simulink model "PCtest_pLBase"  (R2021b)
settings: Solver=FixedStepAuto  StartTime=0.0  StopTime=600  FixedStep=0.005  RelTol=1e-3
libraries: PuppyLibrary x2
settings Model: Creator=kboxi  LastModifiedBy=kboxi

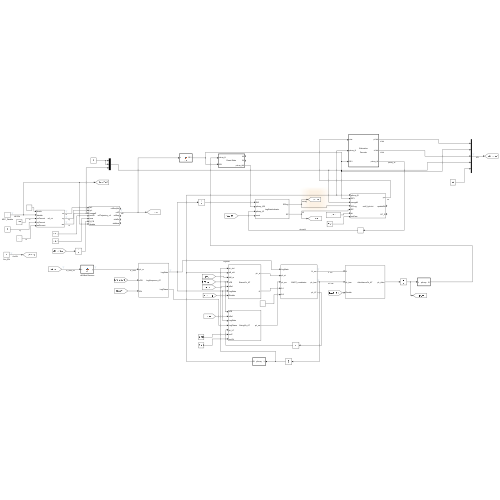
[thumbnail: Simulink's stored preview of the top-level diagram]
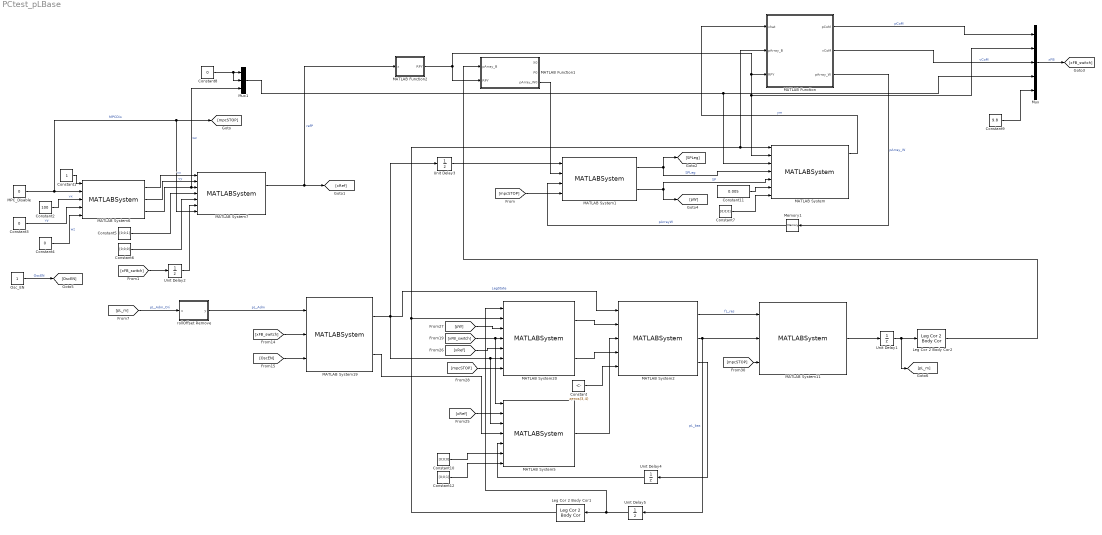
== system PCtest_pLBase ==
  Constant : Constant  Value=zeros(3,4)
  Constant1 : Constant
  Constant10 : Constant  Value=[0;0;0]
  Constant11 : Constant  Value=0.005
  Constant12 : Constant  Value=[0;0;1]
  Constant2 : Constant  Value=100
  Constant3 : Constant  Value=0
  Constant4 : Constant  Value=0
  Constant5 : Constant  Value=[0;0;1]
  Constant6 : Constant  Value=[0;0;0]
  Constant7 : Constant  Value=[0;0;0]
  Constant8 : Constant  Value=0
  Constant9 : Constant  Value=9.8
  Leg Cor 2 Body Cor1 : PuppyLibrary/Leg Cor 2 Body Cor  SystemSampleTime=-1  VariantActivationTime=update diagram  Latency=0  AutoFrameSizeCalculation=off
  Leg Cor 2 Body Cor2 : PuppyLibrary/Leg Cor 2 Body Cor  SystemSampleTime=-1  VariantActivationTime=update diagram  Latency=0  AutoFrameSizeCalculation=off
  MATLAB Function : MATLAB Function  TreatAsAtomicUnit=on
  MATLAB Function1 : MATLAB Function  TreatAsAtomicUnit=on
  MATLAB Function2 : MATLAB Function  TreatAsAtomicUnit=on
  MATLAB System : MATLABSystem  System=estX_byJoint  SimulateUsing=Code generation
      mask Type: estX_byJoint
      mask Display:
      | disp('estX_byJoint');
      | port_label('input',1,'pArray_B');
      | port_label('input',2,'RPY');
      | port_label('input',3,'omegaB');
      | port_label('input',4,'SPLeg');
      | port_label('input',5,'SP');
      | port_label('input',6,'dt');
      | port_label('input',7,'surPara');
      | port_label('output',1,'ym');
      | port_label('output',2,'updateEN');
      | port_label('output',3,'KF_R');
  MATLAB System1 : MATLABSystem  System=LegStateIndicator  SimulateUsing=Code generation
      mask Type: LegStateIndicator
      mask Display:
      | disp('LegStateIndicator');
      | port_label('input',1,'SW');
      | port_label('input',2,'pArray_W0');
      | port_label('input',3,'pArray_W');
      | port_label('input',4,'reset');
      | port_label('output',1,'SPLeg');
      | port_label('output',2,'SP');
  MATLAB System11 : MATLABSystem  System=AdmittanceCtr_AT  lateral_width=0.097  sagetial_width=0.2108  roll_Off=0.037  hIni=0.19  m=3  ks1=21  ks2=21  ks3=21  bs1=0  bs2=0  bs3=0  dt=0.005  SimulateUsing=Interpreted execution
      mask Type: AdmittanceCtr_AT
      mask Display:
      | disp('AdmittanceCtr_AT');
      | port_label('input',1,'fL');
      | port_label('input',2,'pL_bas');
      | port_label('input',3,'Disable');
      | port_label('output',1,'pL_Adm');
  MATLAB System19 : MATLABSystem  System=LegSequence_AT  tSW=0.3  SampleTime=0.005  OffsetTime=0  TickTime=0  startPhase=0  SimulateUsing=Interpreted execution
      mask Type: LegSequence_AT
      mask Display:
      | disp('LegSequence_AT');
      | port_label('input',1,'pL_m');
      | port_label('input',2,'xFB');
      | port_label('input',3,'EN');
      | port_label('output',1,'LegState');
      | port_label('output',2,'LegPhase');
  MATLAB System2 : MATLABSystem  System=SWST_combinator  SimulateUsing=Code generation
      mask Type: SWST_combinator
      mask Display:
      | disp('SWST_combinator');
      | port_label('input',1,'LegState');
      | port_label('input',2,'pL_st');
      | port_label('input',3,'pL_sw');
      | port_label('input',4,'fL1');
      | port_label('input',5,'fL2');
      | port_label('output',1,'fL_res');
      | port_label('output',2,'pL_bas');
      | port_label('output',3,'pL_LF');
  MATLAB System20 : MATLABSystem  System=StanceCtr_AT  tSW=0.3  tSample=0.005  r0=0.19  lateral_width=0.097  sagetial_width=0.2108  roll_Off=0.037  kp=zeros( 1, 6 )  kd=zeros( 1, 6 )  ki=zeros( 1, 6 )  SimulateUsing=Code generation
      mask Type: StanceCtr_AT
      mask Display:
      | disp('StanceCtr_AT');
      | port_label('input',1,'pL_old');
      | port_label('input',2,'pB_old');
      | port_label('input',3,'pW_m');
      | port_label('input',4,'xFB');
      | port_label('input',5,'xRef');
      | port_label('input',6,'LegState');
      | port_label('input',7,'Disable');
      | port_label('output',1,'pL_st');
      | port_label('output',2,'fL');
  MATLAB System5 : MATLABSystem  System=SwingCtr_AT  tSW=0.3  tSample=0.005  r0=[0;0;0.19]  StepH=0.05  lateral_width=0.097  sagetial_width=0.2108  roll_Off=0.037  kx_cv=0  kx_dv=0  ky_cv=0  ky_dv=0  k_wz=0.8  SimulateUsing=Code generation
      mask Type: SwingCtr_AT
      mask Display:
      | disp('SwingCtr_AT');
      | port_label('input',1,'xFB');
      | port_label('input',2,'xRef');
      | port_label('input',3,'LegState');
      | port_label('input',4,'LegPhase');
      | port_label('input',5,'pL_LF');
      | port_label('input',6,'surP');
      | port_label('input',7,'surVN');
      | port_label('output',1,'pL_sw');
  MATLAB System6 : MATLABSystem  System=ref_ctr  vxMax=0.3  vyMax=0.2  wzMax=0.8  SimulateUsing=Code generation
      mask Type: ref_ctr
      mask Display:
      | disp('ref_ctr');
      | port_label('input',1,'timeIn');
      | port_label('input',2,'disable');
      | port_label('input',3,'vxPercent');
      | port_label('input',4,'vyPercent');
      | port_label('input',5,'wzPercent');
      | port_label('output',1,'vx');
      | port_label('output',2,'vy');
      | port_label('output',3,'wz');
  MATLAB System7 : MATLABSystem  System=refTrajectory_v4  r0=[ 0; 0; 0.19 ]  theta0=[ 0; 0; 0 ]  dr0=[ 0; 0; 0 ]  omega0=[ 0; 0; 0 ]  desHeight=0.19  sitaErr_K=[0;0;0]  dt=0.005  numP=6  SimulateUsing=Code generation
      mask Type: refTrajectory_v4
      mask Display:
      | disp('refTrajectory_v4');
      | port_label('input',1,'vxL');
      | port_label('input',2,'vyL');
      | port_label('input',3,'omegaZ');
      | port_label('input',4,'surVN');
      | port_label('input',5,'sura');
      | port_label('input',6,'X_FB');
      | port_label('input',7,'disable');
      | port_label('output',1,'refSeqOut');
      | port_label('output',2,'refP');
      | port_label('output',3,'refSeq');
      | port_label('output',4,'sitaErr');
      | port_label('output',5,'sitaNow');
  MPC_Disable : Constant  Value=0
  Memory1 : Memory  InitialCondition=zeros(12,1)  InheritSampleTime=on
  Mux : Mux  Inputs=5
  Mux1 : Mux  Inputs=3
  Osc_EN : Constant
  Unit Delay1 : UnitDelay  InitialCondition=[0;0;-0.19;0;0;-0.19;0;0;-0.19;0;0;-0.19]*1000  SampleTime=-1  HasFrameUpgradeWarning=on
  Unit Delay2 : UnitDelay  InitialCondition=[0;0;0.19;zeros(9,1);9.8]  SampleTime=-1  HasFrameUpgradeWarning=on
  Unit Delay3 : UnitDelay  InitialCondition=[1;1;1;1]  SampleTime=-1  HasFrameUpgradeWarning=on
  Unit Delay4 : UnitDelay  InitialCondition=[0;0;-0.19;0;0;-0.19;0;0;-0.19;0;0;-0.19]  SampleTime=-1  HasFrameUpgradeWarning=on
  Unit Delay5 : UnitDelay  InitialCondition=[0;0;-0.19;0;0;-0.19;0;0;-0.19;0;0;-0.19]  SampleTime=-1  HasFrameUpgradeWarning=on
  rollOffset Remove : MATLAB Function  TreatAsAtomicUnit=on
  wires:
  [mpcSTOP] -> MATLAB System11/3
  MATLAB System2/1 -> MATLAB System11/1  "fL_res"
  Leg Cor 2 Body Cor1/1 -> MATLAB System20/2, MATLAB Function/2(pArray_B), MATLAB System/1
  Constant/1 -> MATLAB System2/5
  [xFB_switch] -> MATLAB System20/4, MATLAB System5/1
  MATLAB System2/2 -> MATLAB System11/2, Unit Delay5/1  "pL_bas"
  [xRef] -> MATLAB System5/2
  Unit Delay4/1 -> MATLAB System5/5
  MATLAB System2/3 -> Unit Delay4/1
  [OscEN] -> MATLAB System19/3
  MATLAB System20/2 -> MATLAB System2/4
  MATLAB System19/2 -> MATLAB System5/4
  [pW] -> MATLAB System20/3
  Unit Delay5/1 -> MATLAB System20/1, Leg Cor 2 Body Cor1/1
  MATLAB System20/1 -> MATLAB System2/2
  [mpcSTOP] -> MATLAB System20/7
  [xRef] -> MATLAB System20/5
  MATLAB System5/1 -> MATLAB System2/3
  MATLAB System19/1 -> MATLAB System2/1, Unit Delay3/1, MATLAB System20/6, MATLAB System5/3  "LegState"
  MPC_Disable/1 -> [mpcSTOP], MATLAB System7/7, MATLAB System6/2  "MPCDis"
  Constant1/1 -> MATLAB System6/1
  Constant2/1 -> MATLAB System6/3  "vx"
  Constant3/1 -> MATLAB System6/4  "vy"
  Constant4/1 -> MATLAB System6/5  "wz"
  MATLAB System6/1 -> MATLAB System7/1  "vx"
  MATLAB System6/2 -> MATLAB System7/2  "vy"
  MATLAB System6/3 -> Mux1/3, MATLAB System7/3  "wz"
  Constant5/1 -> MATLAB System7/4
  Constant6/1 -> MATLAB System7/5
  Memory1/1 -> MATLAB System1/3  "pArrayW"
  MATLAB Function/3(pArray_W) -> Memory1/1  "pArray_W"
  Constant11/1 -> MATLAB System/6
  MATLAB System1/1 -> [SPLeg], MATLAB System/4  "SPLeg"
  MATLAB System1/2 -> MATLAB System/5, [pW]  "SP"
  [mpcSTOP] -> MATLAB System1/4
  MATLAB System/1 -> MATLAB Function/1(xhat)  "ym"
  MATLAB Function1/3(pArray_W0) -> MATLAB System1/2
  MATLAB System7/2 -> [xRef], MATLAB Function2/1(x)  "refP"
  MATLAB Function2/1(RPY) -> MATLAB Function1/2(RPY), Mux/2, MATLAB System/2, MATLAB Function/3(RPY)
  Constant7/1 -> MATLAB System/7
  MATLAB Function/1(pCoM) -> Mux/1  "pCoM"
  MATLAB Function/2(vCoM) -> Mux/3  "vCoM"
  Constant8/1 -> Mux1/2, Mux1/1
  Mux1/1 -> MATLAB System/3, Mux/4
  Mux/1 -> [xFB_switch]  "xFB"
  Osc_EN/1 -> [OscEN]  "OscEN"
  Unit Delay1/1 -> [pL_m], Leg Cor 2 Body Cor2/1
  MATLAB System11/1 -> Unit Delay1/1
  Leg Cor 2 Body Cor2/1 -> MATLAB Function1/1(pArray_B)
  [xFB_switch] -> Unit Delay2/1
  Unit Delay2/1 -> MATLAB System7/6
  Constant9/1 -> Mux/5
  Constant10/1 -> MATLAB System5/6
  Constant12/1 -> MATLAB System5/7
  [xFB_switch] -> MATLAB System19/2
  Unit Delay3/1 -> MATLAB System1/1
  [pL_m] -> rollOffset Remove/1(u)  "pL_Adm_Ori"
  rollOffset Remove/1(y) -> MATLAB System19/1  "pL_Adm"

== matlab function PCtest_pLBase/rollOffset Remove ==
  data: u input; y output size=[12,1]
function y = fcn(u)
roll_Off=0.037;
tmp = reshape(u,3,4)-[0,0,0,0;
                    roll_Off,-roll_Off,roll_Off,-roll_Off;
                    0,0,0,0]*1000;
y=reshape(tmp,12,1)/1000;

== matlab function PCtest_pLBase/MATLAB Function2 ==
  data: x input; RPY output size=[3,1]
function RPY = fcn(x)
RPY=x(4:6);

== matlab function PCtest_pLBase/MATLAB Function ==
  data: xhat input; pCoM output size=[3,1]; vCoM output size=[3,1]; pArray_B input; RPY input; pArray_W output size=[12,1]
function [pCoM,vCoM,pArray_W] = fcn(xhat,pArray_B,RPY)
% pB the CoM position in the world coordinate
% vB the CoM velocity
% Wpi the foot-end position in the world coordinate
pCoM=[xhat(1);xhat(2);xhat(3)];
vCoM=[xhat(4);xhat(5);xhat(6)];
Rz=[cos(RPY(3)),-sin(RPY(3)),0;
    sin(RPY(3)),cos(RPY(3)),0;
    0,0,1];
Ry=[cos(RPY(2)),0,sin(RPY(2));
    0,1,0;
    -sin(RPY(2)),0,cos(RPY(2))];
Rx=[1,0,0;
    0,cos(RPY(1)),-sin(RPY(1));
    0,sin(RPY(1)),cos(RPY(1))];
R=Rz*Ry*Rx;
pArray_B=reshape(pArray_B,3,4)/1000;
temp=R*pArray_B+pCoM*[1,1,1,1];
pArray_W=[temp(:,1);temp(:,2);temp(:,3);temp(:,4)];

== matlab function PCtest_pLBase/MATLAB Function1 ==
  data: pArray_B input; RPY input; X0 output; P0 output; pArray_W0 output
function [X0,P0,pArray_W0]=fcn(pArray_B,RPY)
% NOTE: pArray_W0 is calculated without the value of yaw angle!!!
Ry=[cos(RPY(2)),0,sin(RPY(2));
    0,1,0;
    -sin(RPY(2)),0,cos(RPY(2))];
Rx=[1,0,0;
    0,cos(RPY(1)),-sin(RPY(1));
    0,sin(RPY(1)),cos(RPY(1))];
pArray_B=reshape(pArray_B,3,4)/1000;
pArray_float=Ry*Rx*pArray_B; % foot-end position in floating coordinate
zOff=-min(pArray_float(3,:));
temp=pArray_float+[0;0;zOff]*[1,1,1,1];
pCoM=[0;0;zOff];
vCoM=[0;0;0];
pArray_W0=[temp(:,1);temp(:,2);temp(:,3);temp(:,4)];
X0=[pCoM;vCoM;zeros(3,1)];
P0=eye(9)*10^-3;
